simulink model "tos_sim"  (Simulink 7.0)
settings: Solver=ode45  StartTime=0.0  StopTime=6  RelTol=1e-3
values from neighbouring files (symbols this model uses):
  r = rlocus(Aol,Bol,Col,Dol,k5)    [fig10_15.m]    (also in fig10_18.m = [0*g;1]; fig10_19.m = [0*g;1]; fig10_20.m = [0*g;1]; fig10_21.m = [0*g;1])
settings Model: Creator=abbas  LastModifiedBy=abbas
settings DataIOCC: SignalLoggingName=sigsOut
settings OptimizationCC: BooleanDataType=off
settings DebuggingCC: SaveWithParameterizedLinksMsg=none  SignalResolutionControl=TryResolveAllWithWarning  SolverPrmCheckMsg=none  MultiTaskDSMMsg=warning  MultiTaskCondExecSysMsg=none  StrictBusMsg=None
settings HardwareCC: TargetUnknown=on
settings RTWCC: IncludeERTFirstTime=on
settings STFCustomTargetCC: GenFloatMathFcnCalls=ANSI_C  ModelReferenceCompliant=off  SystemTargetFile=grt.tlc

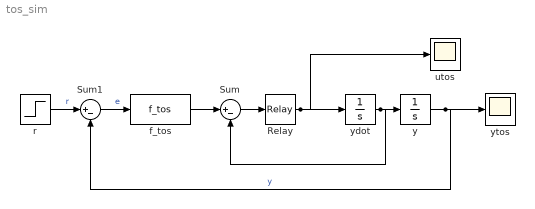
== system tos_sim ==
  " f_tos" : MATLABFcn  MATLABFcn=f_tos  OutputDimensions=1
  " r" : Step  Time=0  After=r  SampleTime=.1
  " ydot" : Integrator
  Relay : Relay  OnSwitchValue=.01  OffSwitchValue=-.01  OffOutputValue=-1  OutDataType=sfix(16)  OutScaling=2^0
  Sum : Sum  Inputs=|+-  OutDataType=sfix(16)  OutScaling=2^0  SaturateOnIntegerOverflow=on  InputSameDT=on
  Sum1 : Sum  Inputs=|+-  OutDataType=sfix(16)  OutScaling=2^0  SaturateOnIntegerOverflow=on  InputSameDT=on
  utos : Scope
      settings: YMin=-1  YMax=1  SaveName=utos  DataFormat=Array
  y : Integrator
  ytos : Scope
      settings: YMin=49.9  YMax=51.1  SaveName=ytos  DataFormat=Array
  wires:
  " ydot"/1 -> Sum/2, y/1
  Sum1/1 -> " f_tos"/1  "e"
  " f_tos"/1 -> Sum/1
  y/1 -> Sum1/2, ytos/1  "y"
  " r"/1 -> Sum1/1  "r"
  Relay/1 -> " ydot"/1, utos/1
  Sum/1 -> Relay/1
